simulink model "State_flow"  (Simulink 9.0)
settings: Solver=VariableStepAuto  StartTime=0.0  StopTime=inf  RelTol=1e-3
settings Model: Creator=yinch  LastModifiedBy=yinch
settings DataIOCC: SaveFormat=Dataset
settings OptimizationCC: LifeSpan=auto
settings DebuggingCC: UnderspecifiedInitializationDetection=Simplified  MergeDetectMultiDrivingBlocksExec=error  SFUnexpectedBacktrackingDiag=error  SFExecutionAtInitializationDiag=warning
settings HardwareCC: ProdBitPerPointer=64  ProdBitPerSizeT=64  ProdBitPerPtrDiffT=64  ProdLargestAtomicFloat=Float  ProdIntDivRoundTo=Zero  ProdEndianess=LittleEndian  ProdWordSize=64  ProdHWDeviceType=Intel->x86-64 (Windows64)
settings ModelReferenceCC: PropagateSignalLabelsOutOfModel=on
settings CodeAppCC: StateflowObjectComments=off
settings GRTTargetCC: TargetLangStandard=C99 (ISO)
settings ConfigComp: CovMetricSettings=dwe  CovHtmlReporting=off  CovSaveCumulativeToWorkspaceVar=off  CovSaveSingleToWorkspaceVar=off  CovExternalEMLEnable=on

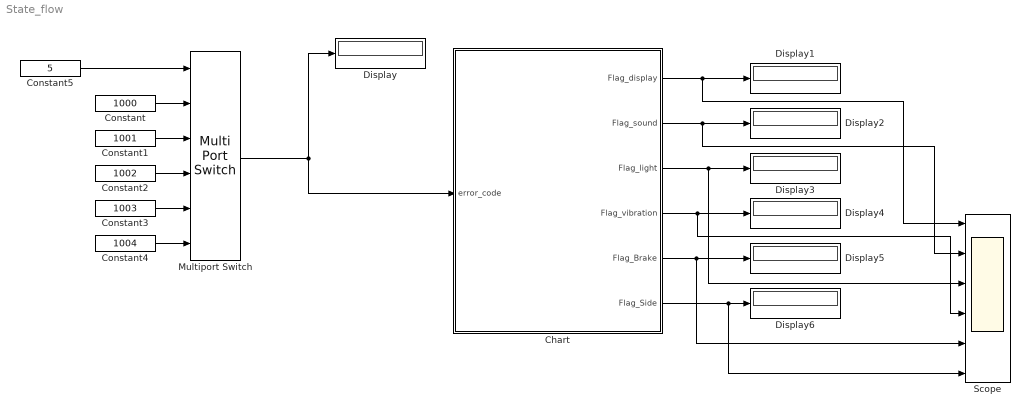
== system State_flow ==
  Chart : Stateflow chart  TreatAsAtomicUnit=on
  Constant : Constant  Value=1000
  Constant1 : Constant  Value=1001
  Constant2 : Constant  Value=1002
  Constant3 : Constant  Value=1003
  Constant4 : Constant  Value=1004
  Constant5 : Constant  Value=5
  Display{,1..6} (7 alike) : Display
  Multiport Switch : MultiPortSwitch  Inputs=5
  Scope : Scope  NumInputPorts=6
  wires:
  Constant/1 -> Multiport Switch/2
  Constant1/1 -> Multiport Switch/3
  Constant2/1 -> Multiport Switch/4
  Constant3/1 -> Multiport Switch/5
  Constant4/1 -> Multiport Switch/6
  Multiport Switch/1 -> Chart/1(error_code), Display/1
  Constant5/1 -> Multiport Switch/1
  Chart/1(Flag_display) -> Scope/1, Display1/1
  Chart/2(Flag_sound) -> Scope/2, Display2/1
  Chart/3(Flag_light) -> Scope/3, Display3/1
  Chart/4(Flag_vibration) -> Scope/4, Display4/1
  Chart/5(Flag_Brake) -> Scope/5, Display5/1
  Chart/6(Flag_Side) -> Scope/6, Display6/1

== stateflow chart Chart ==
  state Normal
    en:Flag_display=0;
    en:Flag_sound=0;
    en:Flag_light=0;
    en:Flag_vibration=0;
    en:Flag_Brake=0;
    en:Flag_Side=0;
  state Tired
    en:Flag_display=1;
    en:Flag_sound=1;
    en:Flag_light=0;
    en:Flag_vibration=0;
    en:Flag_Brake=0;
    en:Flag_Side=0;
  state ZouShen
    en:Flag_display=1;
    en:Flag_sound=1;
    en:Flag_light=1;
    en:Flag_vibration=1;
    en:Flag_Brake=1;
    en:Flag_Side=0
  state Sleep
    en:Flag_display=1;
    en:Flag_sound=2;
    en:Flag_light=2;
    en:Flag_vibration=2;
    en:Flag_Brake=0;
    en:Flag_Side=0
  state Danger
    en:Flag_display=1;
    en:Flag_sound=2;
    en:Flag_light=2;
    en:Flag_vibration=2;
    en:Flag_Brake=0;
    en:Flag_Side=1
  (junction 15) -> Tired : [error_code==1001]
  (junction 17) -> (junction 15) [order 2]
  Tired -> (junction 18) : [error_code~=1001]
  (junction 18) -> Tired [order 2] : [error_code==1001]
  (default) -> (junction 16)
  (junction 16) -> Normal [order 1] : [error_code==1000]
  (junction 16) -> (junction 19) [order 2]
  (junction 17) -> ZouShen [order 1] : [error_code==1002]
  (junction 22) -> (junction 17)
  Normal -> (junction 18) : [error_code~=1000]
  ZouShen -> (junction 18) : [error_code~=1002]
  (junction 18) -> Normal [order 1] : [error_code==1000]
  (junction 18) -> ZouShen [order 3] : [error_code==1002]
  Danger -> (junction 18) : [error_code~=1004]
  (junction 18) -> Sleep [order 4] : [error_code==1003]
  Sleep -> (junction 18) : [error_code~=1003]
  (junction 18) -> Danger [order 5] : [error_code==1004]
  (junction 19) -> Danger [order 1] : [error_code==1004]
  (junction 19) -> (junction 20) [order 2]
  (junction 21) -> Sleep [order 1] : [error_code==1003]
  (junction 20) -> (junction 21)
  (junction 21) -> (junction 22) [order 2]
  data: error_code input double; Flag_display output double; Flag_sound output double; Flag_light output double; Flag_vibration output double; Flag_Brake output double; Flag_Side output double
